simulink model "BrowarModel"  (R2024a)
settings: Solver=ode5  StartTime=0.0  StopTime=inf  FixedStep=0.1  RelTol=1e-3
undefined symbols (not defined in the file or in its folder): localhost, Matrikon, OI
libraries: opclib x24
(part 4 of 9)

== system BrowarModel/System dozowania drozdzy/XT806H ==
  note: Przetwornik pomiarowy
  In : Inport
  FT : Constant  Value=0
  FT_value : Constant  Value=0
  GUIMon : Gain
  Switch : Switch  Threshold=0.5  SaturateOnIntegerOverflow=off  InputSameDT=off
  Out : Outport
  wires:
  FT_value/1 -> Switch/1
  Switch/1 -> GUIMon/1
  FT/1 -> Switch/2
  GUIMon/1 -> Out/1
  In/1 -> Switch/3

== system BrowarModel/System dozowania drozdzy/XT806L ==
  note: Przetwornik pomiarowy
  In : Inport
  FT : Constant  Value=0
  FT_value : Constant  Value=0
  GUIMon : Gain
  Switch : Switch  Threshold=0.5  SaturateOnIntegerOverflow=off  InputSameDT=off
  Out : Outport
  wires:
  In/1 -> Switch/3
  GUIMon/1 -> Out/1
  FT/1 -> Switch/2
  Switch/1 -> GUIMon/1
  FT_value/1 -> Switch/1

== system BrowarModel/System dozowania drozdzy/XV804 ==
  note: Sterowanie
  GUIMon : Gain
  Lokalne : Constant  Value=0
  Wybor : Switch  Threshold=0.5  SaturateOnIntegerOverflow=off  InputSameDT=off
  Out : Outport
  wires:
  GUIMon/1 -> Out/1
  Wybor/1 -> GUIMon/1
  [TrybSter] -> Wybor/2
  [XV804] -> Wybor/1
  Lokalne/1 -> Wybor/3

== system BrowarModel/System dozowania drozdzy/XV806 ==
  note: Sterowanie
  GUIMon : Gain
  Lokalne : Constant  Value=0
  Wybor : Switch  Threshold=0.5  SaturateOnIntegerOverflow=off  InputSameDT=off
  Out : Outport
  wires:
  Lokalne/1 -> Wybor/3
  [XV806] -> Wybor/1
  [TrybSter] -> Wybor/2
  Wybor/1 -> GUIMon/1
  GUIMon/1 -> Out/1

== system BrowarModel/Kadz fermentacyjna/ET704/Zaklocenia pomiarowe ==
  Product1 : Product  InputSameDT=on  RndMeth=Zero  SaturateOnIntegerOverflow=on  OutDataTypeStr=Inherit: Same as first input
  Product3 : Product  InputSameDT=on  RndMeth=Zero  SaturateOnIntegerOverflow=on  OutDataTypeStr=Inherit: Same as first input
  Random Number : RandomNumber  Variance=.5  Seed=4365624  SampleTime=0.1
  Transfer Fcn1 : TransferFcn  Denominator=[0.5 1]
  Transfer Fcn2 : TransferFcn  Denominator=[0.5 1]
  Zaklocenia pomiarowe : Constant  Value=ZakloceniaPom
  Out : Outport
  wires:
  Random Number/1 -> Product3/1
  Product3/1 -> Transfer Fcn1/1
  Transfer Fcn1/1 -> Transfer Fcn2/1
  Transfer Fcn2/1 -> Out/1
  Zaklocenia pomiarowe/1 -> Product1/2
  [ZaklPom] -> Product1/1
  Product1/1 -> Product3/2

== system BrowarModel/Kadz fermentacyjna/ET705/Zaklocenia pomiarowe ==
  Product1 : Product  InputSameDT=on  RndMeth=Zero  SaturateOnIntegerOverflow=on  OutDataTypeStr=Inherit: Same as first input
  Product3 : Product  InputSameDT=on  RndMeth=Zero  SaturateOnIntegerOverflow=on  OutDataTypeStr=Inherit: Same as first input
  Random Number : RandomNumber  Variance=.5  Seed=4365624  SampleTime=0.1
  Transfer Fcn1 : TransferFcn  Denominator=[0.5 1]
  Transfer Fcn2 : TransferFcn  Denominator=[0.5 1]
  Zaklocenia pomiarowe : Constant  Value=ZakloceniaPom
  Out : Outport
  wires:
  Product1/1 -> Product3/2
  [ZaklPom] -> Product1/1
  Zaklocenia pomiarowe/1 -> Product1/2
  Transfer Fcn2/1 -> Out/1
  Transfer Fcn1/1 -> Transfer Fcn2/1
  Product3/1 -> Transfer Fcn1/1
  Random Number/1 -> Product3/1

== system BrowarModel/Kadz fermentacyjna/Kadz fermentacyjna/Kadz ==
  note: Kadz fermentacji
  Doplyw brzeczki : Inport
  Odplyw : Inport  Port=2
  Strumien ciepla : Inport  Port=3
  Temperatura brzeczki : Inport  Port=4
  Wyciek : Inport  Port=5
  Obroty mieszadla : Inport  Port=6
  Gain : Gain  Gain=1/1.5
  Math Function : Math  Operator=sqrt  SignedPower=on
  Max wyciek : Constant  Value=0.1
  Model akumulacji ciepla w zbiorniku z ciecza : Subsystem
  Model rozkladu temperatur : Subsystem
  Model utratu ciepla : Subsystem
  Objetosc : Integrator  InitialCondition=0.001  LimitOutput=on  UpperSaturationLimit=48  LowerSaturationLimit=0.001
  Powierzchnia dna m2 : Constant  Value=16
  Poziom zbiornika : Subsystem
  Product : Product  RndMeth=Zero
  Product1 : Product  RndMeth=Zero
  Sat doplyw (F>=0) : Saturate  UpperLimit=inf  LowerLimit=0
  Sat uszk (F>=0)1 : Saturate  UpperLimit=1  LowerLimit=0
  Sum1 : Sum  Inputs=|+-
  Sum2 : Sum  Inputs=|+-
  Sum4 : Sum  Inputs=|++
  Poziom wysoki : Outport
  Poziom niski : Outport  Port=2
  Poziom : Outport  Port=3
  Temp sensor gorny : Outport  Port=4
  Temp sensor srodkowy : Outport  Port=5
  Temp sensor dolny : Outport  Port=6
  Cieplo odebrane : Outport  Port=7
  Temperatura srednia : Outport  Port=8
  Temp przy dnie : Outport  Port=9
  wires:
  Model rozkladu temperatur/1(Temperatura lustra zbiornika) -> Model utratu ciepla/4(Temperatura lustra)  "dec C"
  Model utratu ciepla/1(Strumien ciepla) -> Model akumulacji ciepla w zbiorniku z ciecza/5(Strumien cieplo traconego)
  Sat doplyw (F>=0)/1 -> Sum1/1, Model akumulacji ciepla w zbiorniku z ciecza/3(Strumien doplywu cieczy)  "m3/s"
  Model akumulacji ciepla w zbiorniku z ciecza/2(Srednia temperaturacie czy) -> Model rozkladu temperatur/2(Srednia temperatura), Model utratu ciepla/3(Srednia temperatura), Temperatura srednia/1
  Powierzchnia dna m2/1 -> Model utratu ciepla/2(Pole podstawy zbiornika), Poziom zbiornika/2(Powierzchnia dna)  "m2"
  Objetosc/1 -> Model akumulacji ciepla w zbiorniku z ciecza/1(Objetosc cieczy w zbiorniku), Poziom zbiornika/1(Objetosc)  "m3"
  Poziom zbiornika/3(Poziom) -> Model utratu ciepla/1(Poziom), Poziom/1, Model rozkladu temperatur/1(Poziom), Gain/1
  Sum2/1 -> Objetosc/1
  Sum1/1 -> Sum2/1
  Model akumulacji ciepla w zbiorniku z ciecza/1(Srumien cieczy odparowanej) -> Sum2/2  "m3/s"
  Poziom zbiornika/1(Poziom  wysoki) -> Poziom wysoki/1
  Doplyw brzeczki/1 -> Sat doplyw (F>=0)/1
  Poziom zbiornika/2(Poziom niski) -> Poziom niski/1
  Model rozkladu temperatur/2(Sensor temperatury gorny) -> Temp sensor gorny/1
  Model rozkladu temperatur/3(Sensor temperatury srodkowy) -> Temp sensor srodkowy/1
  Model rozkladu temperatur/4(Sensor temperatury dolny) -> Temp sensor dolny/1
  Obroty mieszadla/1 -> Model rozkladu temperatur/3(Obroty mieszadla)
  Strumien ciepla/1 -> Model akumulacji ciepla w zbiorniku z ciecza/4(Strumien cieplna dostepny)
  Model rozkladu temperatur/5(Temperatura przy dnie zbiornika) -> Temp przy dnie/1
  Model akumulacji ciepla w zbiorniku z ciecza/3(Strumien ciepla odebrany) -> Cieplo odebrane/1
  Temperatura brzeczki/1 -> Model akumulacji ciepla w zbiorniku z ciecza/6(Temperatura strumien doplywu cieczy)
  Odplyw/1 -> Sum4/1  "m3/h"
  Wyciek/1 -> Sat uszk (F>=0)1/1
  Product/1 -> Sum4/2
  Sat uszk (F>=0)1/1 -> Product/1
  Product1/1 -> Product/2
  Max wyciek/1 -> Product1/1  "m3/s"
  Math Function/1 -> Product1/2
  Gain/1 -> Math Function/1
  Sum4/1 -> Sum1/2, Model akumulacji ciepla w zbiorniku z ciecza/2(Strumien odplywu cieczy)

== system BrowarModel/Kadz fermentacyjna/Kadz fermentacyjna/Model mieszadla ==
  Poziom : Inport
  Obroty : Inport  Port=2
  " Redukcja obrotow" : Gain  Gain=1/720
  " Redukcja obrotow1" : Gain  Gain=1/4
  Dot Product : DotProduct  OutDataTypeStr=Inherit: Inherit via internal rule
  Math Function : Math  Operator=square  SignedPower=on
  Sat FS : Saturate  UpperLimit=1  LowerLimit=0
  Wplyw stopnia wypelnienia na obciazenie : Lookup  InputValues=[0,0.3,1,2]  Table=[0.1,0.1,1,1]  SaturateOnIntegerOverflow=off
  Obroty zredukowane : Outport
  Obciazenie : Outport  Port=2
  wires:
  Obroty/1 -> " Redukcja obrotow"/1  "obr/min"
  " Redukcja obrotow"/1 -> Math Function/1, Obroty zredukowane/1  "obr/min"
  Poziom/1 -> Wplyw stopnia wypelnienia na obciazenie/1
  Math Function/1 -> " Redukcja obrotow1"/1
  " Redukcja obrotow1"/1 -> Dot Product/1
  Wplyw stopnia wypelnienia na obciazenie/1 -> Dot Product/2
  Dot Product/1 -> Sat FS/1
  Sat FS/1 -> Obciazenie/1

== system BrowarModel/Kadz fermentacyjna/Kadz fermentacyjna/Model ogrzewacza ==
  note: Ogrzewacz elektryczny
  note: Uszkodzenie ogrzewacza
  Sterowanie : Inport
  Spadek mocy : Inport  Port=2
  Const : Constant  Value=100
  GUIMon : Gain
  Gain : Gain  Gain=1/100
  Gain1 : Gain  Gain=1/100
  Maksymalna moc : Constant  Value=10000000
  Product : Product  RndMeth=Zero
  Product1 : Product  RndMeth=Zero
  Quantizer : Quantizer  QuantizationInterval=20
  Sat ster : Saturate  UpperLimit=100  LowerLimit=0
  Sat uszk : Saturate  UpperLimit=100  LowerLimit=0
  Sat zero : Saturate  UpperLimit=inf  LowerLimit=0
  Sum1 : Sum  Inputs=|+-
  Sum2 : Sum  Inputs=|+-
  Transfer Fcn : TransferFcn  Denominator=[60 1]
  Transfer Fcn1 : TransferFcn  Denominator=[60 1]
  Zaklocenia : Subsystem
  Cieplo dostarczone : Outport
  wires:
  Sat ster/1 -> Quantizer/1
  Sterowanie/1 -> Sat ster/1
  Quantizer/1 -> GUIMon/1
  Gain/1 -> Product/1
  Zaklocenia/1(Out) -> Sum1/2
  Product/1 -> Transfer Fcn/1
  Transfer Fcn/1 -> Transfer Fcn1/1
  Sum1/1 -> Sat zero/1
  Transfer Fcn1/1 -> Sum1/1, Zaklocenia/1(In)
  GUIMon/1 -> Gain/1
  Sat zero/1 -> Cieplo dostarczone/1
  Maksymalna moc/1 -> Product1/1
  Product1/1 -> Product/2
  Spadek mocy/1 -> Sat uszk/1
  Sat uszk/1 -> Sum2/2
  Sum2/1 -> Gain1/1
  Const/1 -> Sum2/1
  Gain1/1 -> Product1/2

== system BrowarModel/Kadz fermentacyjna/Kadz fermentacyjna/Odplyw z kadzi ==
  note: Doplyw kadzi
  Sterowanie zaworu : Inport
  Przeciek zaworu : Inport  Port=2
  Dlawienie zaworu : Inport  Port=3
  Wyciek : Inport  Port=4
  Poziom w kadzi : Inport  Port=5
  Zalaczenie pompy : Inport  Port=6
  Sterowanie pompy : Inport  Port=7
  Uszkodzenie pompy : Inport  Port=8
  Charakterystyka pompy : Lookup  InputValues="[0\t125\t250\t375\t500\t625\t750\t875\t1000\t1125\t1250\t1375\t1500 1625]"  Table=|  SaturateOnIntegerOverflow=off
      | [0 50	125	178	220	250	270	288	300	310	315	320	323	327
      | ]
  Gain : Gain  Gain=1/100
  Obciazenie silnika : Gain  Gain=1/500
  Product : Product  RndMeth=Zero
  Product1 : Product  RndMeth=Zero
  Relay : Relay  OnOutputValue=0  OffOutputValue=1
  Relay1 : Relay
  Sat uszk : Saturate  UpperLimit=100  LowerLimit=0
  Silnik elektryczny : Subsystem
  "Sterowanie " : DotProduct  OutDataTypeStr=Inherit: Inherit via internal rule
  Straty pompy : Gain  Gain=50/0.15
  Sum : Sum  Inputs=|+-
  Sum1 : Sum  Inputs=|+-
  Wplyw stopnia wypelnienia kadzi : Lookup  InputValues=[-1, 0, 0.05, 1]  Table=[0, 0, 1,1]  SaturateOnIntegerOverflow=off
  Wplyw uszkodzenia : Product  RndMeth=Zero
  Zawor dyskretny : Subsystem
  Przeplyw_wyciek : Outport
  Przeplyw : Outport  Port=2
  Obroty : Outport  Port=3
  Prad silnika : Outport  Port=4
  Silnik Idle : Outport  Port=5
  Silnik Running : Outport  Port=6
  Silnik Alarm : Outport  Port=7
  wires:
  Wplyw stopnia wypelnienia kadzi/1 -> Product/1  "[0,1]"
  Zawor dyskretny/1(Przeplyw) -> Sum1/1, Straty pompy/1, Product1/1
  Dlawienie zaworu/1 -> Zawor dyskretny/4(Dlawienie)
  Poziom w kadzi/1 -> Wplyw stopnia wypelnienia kadzi/1  "m"
  Zalaczenie pompy/1 -> Relay1/1, Silnik elektryczny/1(Zalaczenie)
  Uszkodzenie pompy/1 -> Relay/1, Silnik elektryczny/4(Uszkodzenie)
  Relay/1 -> Wplyw uszkodzenia/2
  Silnik elektryczny/1(Obroty) -> Charakterystyka pompy/1, Obroty/1
  Wplyw uszkodzenia/1 -> Product/2
  Charakterystyka pompy/1 -> "Sterowanie "/2  "kPa"
  "Sterowanie "/1 -> Wplyw uszkodzenia/1
  Relay1/1 -> "Sterowanie "/1
  Product/1 -> Sum/1, Obciazenie silnika/1
  Sum/1 -> Zawor dyskretny/2(Cisnienie)
  Straty pompy/1 -> Sum/2
  Wyciek/1 -> Sat uszk/1
  Product1/1 -> Przeplyw_wyciek/1, Sum1/2
  Sum1/1 -> Przeplyw/1
  Sat uszk/1 -> Gain/1
  Przeciek zaworu/1 -> Zawor dyskretny/3(Przeciek)
  Sterowanie zaworu/1 -> Zawor dyskretny/1(Sterowanie)
  Gain/1 -> Product1/2
  Silnik elektryczny/2(Prad) -> Prad silnika/1
  Silnik elektryczny/3(Idle) -> Silnik Idle/1
  Silnik elektryczny/4(Running) -> Silnik Running/1
  Silnik elektryczny/5(Alarm) -> Silnik Alarm/1
  Sterowanie pompy/1 -> Silnik elektryczny/2(Zadane obroty)
  Obciazenie silnika/1 -> Silnik elektryczny/3(Obciazenie zew)

== system BrowarModel/Kadz fermentacyjna/Kadz fermentacyjna/Silnik elektryczny ==
  note: Uszkodzenie silnika
  note: Silnik elektryczny
  Zalaczenie : Inport
  Zadane obroty : Inport  Port=2
  Obciazenie zew : Inport  Port=3
  Uszkodzenie : Inport  Port=4
  Abs : Abs  SaturateOnIntegerOverflow=off
  Add : Sum
  Add1 : Sum  Inputs=+-
  Const : Constant
  Gain : Gain
  "Hz -> obr/min" : Gain  Gain=60/2
  Inercja mechaniczna : TransferFcn  Denominator=[1 1]
  Poslizg : DotProduct  OutDataTypeStr=Inherit: Inherit via internal rule
  Poslizg jalowy : Constant  Value=0.04
  Poslizg od obciazenia : Gain  Gain=0.05
  Prad jalowy : Gain  Gain=0.5
  Prad nominalny (10A) : Constant  Value=10
  Relay : Relay  OnOutputValue=0  OffOutputValue=1
  Saturation [0,1] : Saturate  UpperLimit=1  LowerLimit=0
  "Saturation [0,1] " : Saturate  UpperLimit=1  LowerLimit=0
  Stan : Subsystem
  Sterowanie : Subsystem
  Sterownik : Subsystem
  Sum : Sum  Inputs=|+-
  Sum1 : Sum  Inputs=|++
  Sum2 : Sum  Inputs=|+-
  Sum3 : Sum  Inputs=|++
  Wplyw uszkodzenia : DotProduct  OutDataTypeStr=Inherit: Inherit via internal rule
  Wplyw obciazenia : DotProduct  OutDataTypeStr=Inherit: Inherit via internal rule
  Wplyw obrotow : DotProduct  OutDataTypeStr=Inherit: Inherit via internal rule
  Zaklocenia : Subsystem
  Zalaczony : DotProduct  OutDataTypeStr=Inherit: Inherit via internal rule
  "obr/min -> FS  " : Gain  Gain=1/1500
  "obr/min -> Hz" : Gain  Gain=1/60*2
  Obroty : Outport
  Prad : Outport  Port=2
  Idle : Outport  Port=3
  Running : Outport  Port=4
  Alarm : Outport  Port=5
  wires:
  Zaklocenia/1(Out) -> Sum2/2
  Sum2/1 -> Sum/1, Add1/1
  Stan/3(Alarm) -> Alarm/1
  Stan/2(Running) -> Zalaczony/2, Running/1
  Stan/1(Idle) -> Idle/1
  Zadane obroty/1 -> Sterowanie/1(Zadane obroty)
  Zalaczony/1 -> Wplyw obrotow/2
  Sum1/1 -> Zalaczony/1  "A"
  Wplyw obrotow/1 -> Prad/1  "A"
  Wplyw uszkodzenia/1 -> "Hz -> obr/min"/1
  Relay/1 -> Stan/2(Zdatny), Wplyw uszkodzenia/2
  Sterownik/1(CV) -> Wplyw uszkodzenia/1
  Uszkodzenie/1 -> Relay/1
  Gain/1 -> "Saturation [0,1] "/1
  Sterowanie/1(Sterowanie) -> Sterownik/2(SP)
  Zalaczenie/1 -> Stan/1(Zalaczony), Sterowanie/2(Zalaczenie)
  "Saturation [0,1] "/1 -> Add/1
  "obr/min -> FS  "/1 -> Gain/1
  Add1/1 -> "obr/min -> FS  "/1
  Add/1 -> Abs/1, Poslizg od obciazenia/1  "FS"
  Saturation [0,1]/1 -> Add/2
  "obr/min -> Hz"/1 -> Sterownik/1(PV)
  Const/1 -> Wplyw obrotow/1
  Abs/1 -> Wplyw obciazenia/1  "FS"
  Wplyw obciazenia/1 -> Sum1/1
  Prad jalowy/1 -> Wplyw obciazenia/2, Sum1/2
  Prad nominalny (10A)/1 -> Prad jalowy/1  "A"
  Poslizg jalowy/1 -> Sum3/2
  Obciazenie zew/1 -> Saturation [0,1]/1  "FS"
  Poslizg od obciazenia/1 -> Sum3/1
  Sum3/1 -> Poslizg/2
  Poslizg/1 -> Sum/2
  "Hz -> obr/min"/1 -> Zaklocenia/1(In), Sum2/1  "[obr/min]"
  Sum/1 -> Inercja mechaniczna/1
  Inercja mechaniczna/1 -> "obr/min -> Hz"/1, Add1/2, Poslizg/1, Obroty/1

== system BrowarModel/Kadz fermentacyjna/LT701/Zaklocenia pomiarowe ==
  Product1 : Product  InputSameDT=on  RndMeth=Zero  SaturateOnIntegerOverflow=on  OutDataTypeStr=Inherit: Same as first input
  Product3 : Product  InputSameDT=on  RndMeth=Zero  SaturateOnIntegerOverflow=on  OutDataTypeStr=Inherit: Same as first input
  Random Number : RandomNumber  Variance=.5  Seed=4365624  SampleTime=0.1
  Transfer Fcn1 : TransferFcn  Denominator=[0.5 1]
  Transfer Fcn2 : TransferFcn  Denominator=[0.5 1]
  Zaklocenia pomiarowe : Constant  Value=ZakloceniaPom
  Out : Outport
  wires:
  Product1/1 -> Product3/2
  [ZaklPom] -> Product1/1
  Zaklocenia pomiarowe/1 -> Product1/2
  Transfer Fcn2/1 -> Out/1
  Transfer Fcn1/1 -> Transfer Fcn2/1
  Product3/1 -> Transfer Fcn1/1
  Random Number/1 -> Product3/1

== system BrowarModel/Kadz fermentacyjna/ST704/Zaklocenia pomiarowe ==
  Product1 : Product  InputSameDT=on  RndMeth=Zero  SaturateOnIntegerOverflow=on  OutDataTypeStr=Inherit: Same as first input
  Product3 : Product  InputSameDT=on  RndMeth=Zero  SaturateOnIntegerOverflow=on  OutDataTypeStr=Inherit: Same as first input
  Random Number : RandomNumber  Variance=.5  Seed=4365624  SampleTime=0.1
  Transfer Fcn1 : TransferFcn  Denominator=[0.5 1]
  Transfer Fcn2 : TransferFcn  Denominator=[0.5 1]
  Zaklocenia pomiarowe : Constant  Value=ZakloceniaPom
  Out : Outport
  wires:
  Product1/1 -> Product3/2
  [ZaklPom] -> Product1/1
  Zaklocenia pomiarowe/1 -> Product1/2
  Transfer Fcn2/1 -> Out/1
  Transfer Fcn1/1 -> Transfer Fcn2/1
  Product3/1 -> Transfer Fcn1/1
  Random Number/1 -> Product3/1

== system BrowarModel/Kadz fermentacyjna/ST705/Zaklocenia pomiarowe ==
  Product1 : Product  InputSameDT=on  RndMeth=Zero  SaturateOnIntegerOverflow=on  OutDataTypeStr=Inherit: Same as first input
  Product3 : Product  InputSameDT=on  RndMeth=Zero  SaturateOnIntegerOverflow=on  OutDataTypeStr=Inherit: Same as first input
  Random Number : RandomNumber  Variance=.5  Seed=4365624  SampleTime=0.1
  Transfer Fcn1 : TransferFcn  Denominator=[0.5 1]
  Transfer Fcn2 : TransferFcn  Denominator=[0.5 1]
  Zaklocenia pomiarowe : Constant  Value=ZakloceniaPom
  Out : Outport
  wires:
  Random Number/1 -> Product3/1
  Product3/1 -> Transfer Fcn1/1
  Transfer Fcn1/1 -> Transfer Fcn2/1
  Transfer Fcn2/1 -> Out/1
  Zaklocenia pomiarowe/1 -> Product1/2
  [ZaklPom] -> Product1/1
  Product1/1 -> Product3/2

== system BrowarModel/Kadz fermentacyjna/TT702H/Zaklocenia pomiarowe ==
  Product1 : Product  InputSameDT=on  RndMeth=Zero  SaturateOnIntegerOverflow=on  OutDataTypeStr=Inherit: Same as first input
  Product3 : Product  InputSameDT=on  RndMeth=Zero  SaturateOnIntegerOverflow=on  OutDataTypeStr=Inherit: Same as first input
  Random Number : RandomNumber  Variance=.5  Seed=4365624  SampleTime=0.1
  Transfer Fcn1 : TransferFcn  Denominator=[0.5 1]
  Transfer Fcn2 : TransferFcn  Denominator=[0.5 1]
  Zaklocenia pomiarowe : Constant  Value=ZakloceniaPom
  Out : Outport
  wires:
  Random Number/1 -> Product3/1
  Product3/1 -> Transfer Fcn1/1
  Transfer Fcn1/1 -> Transfer Fcn2/1
  Transfer Fcn2/1 -> Out/1
  Zaklocenia pomiarowe/1 -> Product1/2
  [ZaklPom] -> Product1/1
  Product1/1 -> Product3/2

== system BrowarModel/Kadz fermentacyjna/TT702L/Zaklocenia pomiarowe ==
  Product1 : Product  InputSameDT=on  RndMeth=Zero  SaturateOnIntegerOverflow=on  OutDataTypeStr=Inherit: Same as first input
  Product3 : Product  InputSameDT=on  RndMeth=Zero  SaturateOnIntegerOverflow=on  OutDataTypeStr=Inherit: Same as first input
  Random Number : RandomNumber  Variance=.5  Seed=4365624  SampleTime=0.1
  Transfer Fcn1 : TransferFcn  Denominator=[0.5 1]
  Transfer Fcn2 : TransferFcn  Denominator=[0.5 1]
  Zaklocenia pomiarowe : Constant  Value=ZakloceniaPom
  Out : Outport
  wires:
  Random Number/1 -> Product3/1
  Product3/1 -> Transfer Fcn1/1
  Transfer Fcn1/1 -> Transfer Fcn2/1
  Transfer Fcn2/1 -> Out/1
  Zaklocenia pomiarowe/1 -> Product1/2
  [ZaklPom] -> Product1/1
  Product1/1 -> Product3/2

== system BrowarModel/Kadz fermentacyjna/TT702M/Zaklocenia pomiarowe ==
  Product1 : Product  InputSameDT=on  RndMeth=Zero  SaturateOnIntegerOverflow=on  OutDataTypeStr=Inherit: Same as first input
  Product3 : Product  InputSameDT=on  RndMeth=Zero  SaturateOnIntegerOverflow=on  OutDataTypeStr=Inherit: Same as first input
  Random Number : RandomNumber  Variance=.5  Seed=4365624  SampleTime=0.1
  Transfer Fcn1 : TransferFcn  Denominator=[0.5 1]
  Transfer Fcn2 : TransferFcn  Denominator=[0.5 1]
  Zaklocenia pomiarowe : Constant  Value=ZakloceniaPom
  Out : Outport
  wires:
  Product1/1 -> Product3/2
  [ZaklPom] -> Product1/1
  Zaklocenia pomiarowe/1 -> Product1/2
  Transfer Fcn2/1 -> Out/1
  Transfer Fcn1/1 -> Transfer Fcn2/1
  Product3/1 -> Transfer Fcn1/1
  Random Number/1 -> Product3/1

== system BrowarModel/Kadz filtracji/ET302/Zaklocenia pomiarowe ==
  Product1 : Product  InputSameDT=on  RndMeth=Zero  SaturateOnIntegerOverflow=on  OutDataTypeStr=Inherit: Same as first input
  Product3 : Product  InputSameDT=on  RndMeth=Zero  SaturateOnIntegerOverflow=on  OutDataTypeStr=Inherit: Same as first input
  Random Number : RandomNumber  Variance=.5  Seed=4365624  SampleTime=0.1
  Transfer Fcn1 : TransferFcn  Denominator=[0.5 1]
  Transfer Fcn2 : TransferFcn  Denominator=[0.5 1]
  Zaklocenia pomiarowe : Constant  Value=ZakloceniaPom
  Out : Outport
  wires:
  Random Number/1 -> Product3/1
  Product3/1 -> Transfer Fcn1/1
  Transfer Fcn1/1 -> Transfer Fcn2/1
  Transfer Fcn2/1 -> Out/1
  Zaklocenia pomiarowe/1 -> Product1/2
  [ZaklPom] -> Product1/1
  Product1/1 -> Product3/2

== system BrowarModel/Kadz filtracji/ET304/Zaklocenia pomiarowe ==
  Product1 : Product  InputSameDT=on  RndMeth=Zero  SaturateOnIntegerOverflow=on  OutDataTypeStr=Inherit: Same as first input
  Product3 : Product  InputSameDT=on  RndMeth=Zero  SaturateOnIntegerOverflow=on  OutDataTypeStr=Inherit: Same as first input
  Random Number : RandomNumber  Variance=.5  Seed=4365624  SampleTime=0.1
  Transfer Fcn1 : TransferFcn  Denominator=[0.5 1]
  Transfer Fcn2 : TransferFcn  Denominator=[0.5 1]
  Zaklocenia pomiarowe : Constant  Value=ZakloceniaPom
  Out : Outport
  wires:
  Product1/1 -> Product3/2
  [ZaklPom] -> Product1/1
  Zaklocenia pomiarowe/1 -> Product1/2
  Transfer Fcn2/1 -> Out/1
  Transfer Fcn1/1 -> Transfer Fcn2/1
  Product3/1 -> Transfer Fcn1/1
  Random Number/1 -> Product3/1

== system BrowarModel/Kadz filtracji/ET307/Zaklocenia pomiarowe ==
  Product1 : Product  InputSameDT=on  RndMeth=Zero  SaturateOnIntegerOverflow=on  OutDataTypeStr=Inherit: Same as first input
  Product3 : Product  InputSameDT=on  RndMeth=Zero  SaturateOnIntegerOverflow=on  OutDataTypeStr=Inherit: Same as first input
  Random Number : RandomNumber  Variance=.5  Seed=4365624  SampleTime=0.1
  Transfer Fcn1 : TransferFcn  Denominator=[0.5 1]
  Transfer Fcn2 : TransferFcn  Denominator=[0.5 1]
  Zaklocenia pomiarowe : Constant  Value=ZakloceniaPom
  Out : Outport
  wires:
  Product1/1 -> Product3/2
  [ZaklPom] -> Product1/1
  Zaklocenia pomiarowe/1 -> Product1/2
  Transfer Fcn2/1 -> Out/1
  Transfer Fcn1/1 -> Transfer Fcn2/1
  Product3/1 -> Transfer Fcn1/1
  Random Number/1 -> Product3/1

== system BrowarModel/Kadz filtracji/Kadz filtracji/Doplyw kadzi ==
  note: Doplyw kadzi
  Sterowanie zaworu : Inport
  Przeciek zaworu : Inport  Port=2
  Dlawienie zaworu : Inport  Port=3
  Wyciek : Inport  Port=4
  Poziom w kadzi zaciernej : Inport  Port=5
  Zalaczenie pompy : Inport  Port=6
  Sterowanie pompy : Inport  Port=7
  Uszkodzenie pompy : Inport  Port=8
  Przepelnienire zb gorny : Inport  Port=9
  Charakterystyka pompy : Lookup  InputValues="[0\t125\t250\t375\t500\t625\t750\t875\t1000\t1125\t1250\t1375\t1500 1625]"  Table=|  SaturateOnIntegerOverflow=off
      | [0 50	125	178	220	250	270	288	300	310	315	320	323	327
      | ]
  Constant : Constant  Value=0
  Gain : Gain  Gain=1/100
  Obciazenie silnika : Gain  Gain=1/500
  Product : Product  RndMeth=Zero
  Product1 : Product  RndMeth=Zero
  Relay : Relay  OnOutputValue=0  OffOutputValue=1
  Relay1 : Relay
  Sat uszk : Saturate  UpperLimit=100  LowerLimit=0
  Silnik elektryczny : Subsystem
  "Sterowanie " : DotProduct  OutDataTypeStr=Inherit: Inherit via internal rule
  Straty pompy : Gain  Gain=50/0.15
  Sum : Sum  Inputs=|+-
  Sum1 : Sum  Inputs=|+-
  Switch : Switch  Threshold=0.5  SaturateOnIntegerOverflow=off  InputSameDT=off
  Wplyw stopnia wypelnienia kadzi zaciernej : Lookup  InputValues=[-1, 0, 0.001, 0.05, 1]  Table=[0, 0, 0, 1, 1]  SaturateOnIntegerOverflow=off
  Wplyw uszkodzenia : Product  RndMeth=Zero
  Zawor dyskretny : Subsystem
  Przeplyw : Outport
  Przeplyw_wyciek : Outport  Port=2
  Obroty : Outport  Port=3
  Prad silnika : Outport  Port=4
  Silnik Idle : Outport  Port=5
  Silnik Running : Outport  Port=6
  Silnik Alarm : Outport  Port=7
  wires:
  Wplyw stopnia wypelnienia kadzi zaciernej/1 -> Product/1  "[0,1]"
  Zawor dyskretny/1(Przeplyw) -> Sum1/1, Straty pompy/1, Product1/1
  Dlawienie zaworu/1 -> Zawor dyskretny/4(Dlawienie)
  Poziom w kadzi zaciernej/1 -> Wplyw stopnia wypelnienia kadzi zaciernej/1  "m"
  Zalaczenie pompy/1 -> Relay1/1, Silnik elektryczny/1(Zalaczenie)
  Uszkodzenie pompy/1 -> Relay/1, Silnik elektryczny/4(Uszkodzenie)
  Relay/1 -> Wplyw uszkodzenia/2
  Silnik elektryczny/1(Obroty) -> Charakterystyka pompy/1, Obroty/1
  Wplyw uszkodzenia/1 -> Product/2
  Charakterystyka pompy/1 -> "Sterowanie "/2  "kPa"
  "Sterowanie "/1 -> Wplyw uszkodzenia/1
  Relay1/1 -> "Sterowanie "/1
  Product/1 -> Sum/1, Obciazenie silnika/1
  Sum/1 -> Zawor dyskretny/2(Cisnienie)
  Straty pompy/1 -> Sum/2
  Wyciek/1 -> Sat uszk/1
  Product1/1 -> Przeplyw_wyciek/1, Sum1/2
  Sat uszk/1 -> Gain/1
  Przeciek zaworu/1 -> Zawor dyskretny/3(Przeciek)
  Sterowanie zaworu/1 -> Zawor dyskretny/1(Sterowanie)
  Gain/1 -> Product1/2
  Silnik elektryczny/2(Prad) -> Prad silnika/1
  Silnik elektryczny/3(Idle) -> Silnik Idle/1
  Silnik elektryczny/4(Running) -> Silnik Running/1
  Silnik elektryczny/5(Alarm) -> Silnik Alarm/1
  Sterowanie pompy/1 -> Silnik elektryczny/2(Zadane obroty)
  Obciazenie silnika/1 -> Silnik elektryczny/3(Obciazenie zew)
  Przepelnienire zb gorny/1 -> Switch/2
  Constant/1 -> Switch/1
  Sum1/1 -> Switch/3
  Switch/1 -> Przeplyw/1

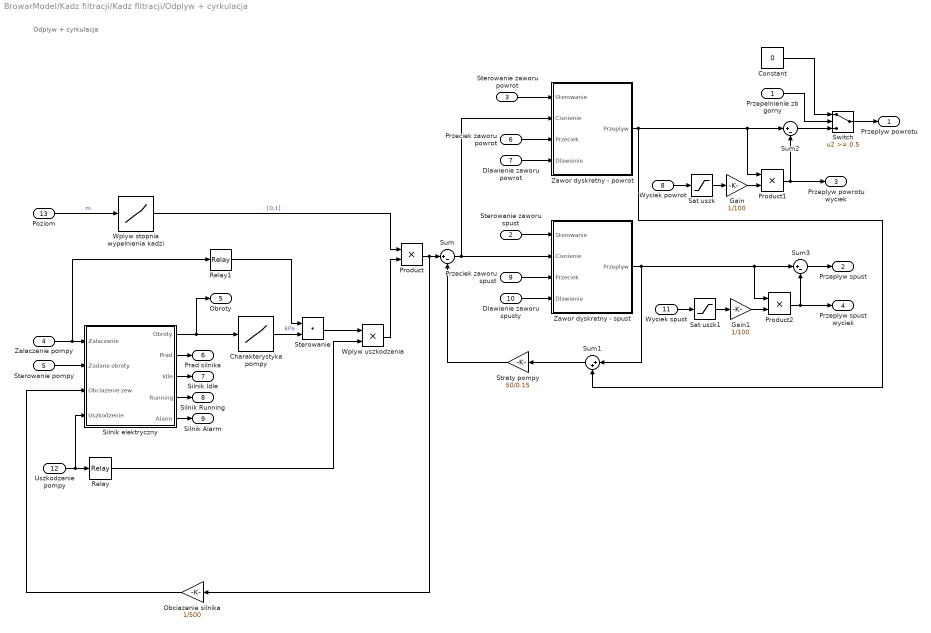
== system BrowarModel/Kadz filtracji/Kadz filtracji/Odplyw + cyrkulacja ==
  note: Odplyw + cyrkulacja
  Przepelnienie zb gorny : Inport
  Sterowanie zaworu spust : Inport  Port=2
  Sterowanie zaworu powrot : Inport  Port=3
  Zalaczenie pompy : Inport  Port=4
  Sterowanie pompy : Inport  Port=5
  Przeciek zaworu powrot : Inport  Port=6
  Dlawienie zaworu powrot : Inport  Port=7
  Wyciek powrot : Inport  Port=8
  Przeciek zaworu spust : Inport  Port=9
  Dlawienie zaworu spusty : Inport  Port=10
  Wyciek spust : Inport  Port=11
  Uszkodzenie pompy : Inport  Port=12
  Poziom : Inport  Port=13
  Charakterystyka pompy : Lookup  InputValues="[0\t125\t250\t375\t500\t625\t750\t875\t1000\t1125\t1250\t1375\t1500 1625]"  Table=|  SaturateOnIntegerOverflow=off
      | [0 50	125	178	220	250	270	288	300	310	315	320	323	327
      | ]
  Constant : Constant  Value=0
  Gain : Gain  Gain=1/100
  Gain1 : Gain  Gain=1/100
  Obciazenie silnika : Gain  Gain=1/500
  Product : Product  RndMeth=Zero
  Product1 : Product  RndMeth=Zero
  Product2 : Product  RndMeth=Zero
  Relay : Relay  OnOutputValue=0  OffOutputValue=1
  Relay1 : Relay
  Sat uszk : Saturate  UpperLimit=100  LowerLimit=0
  Sat uszk1 : Saturate  UpperLimit=100  LowerLimit=0
  Silnik elektryczny : Subsystem
  "Sterowanie " : DotProduct  OutDataTypeStr=Inherit: Inherit via internal rule
  Straty pompy : Gain  Gain=50/0.15
  Sum : Sum  Inputs=|+-
  Sum1 : Sum  Inputs=|++
  Sum2 : Sum  Inputs=|+-
  Sum3 : Sum  Inputs=|+-
  Switch : Switch  Threshold=0.5  SaturateOnIntegerOverflow=off  InputSameDT=off
  Wplyw stopnia wypelnienia kadzi : Lookup  InputValues=[-1, 0, 0.001 0.05, 1]  Table=[0, 0, 0, 1,1]  SaturateOnIntegerOverflow=off
  Wplyw uszkodzenia : Product  RndMeth=Zero
  Zawor dyskretny - powrot : Subsystem
  Zawor dyskretny - spust : Subsystem
  Przeplyw powrotu : Outport
  Przeplyw spust : Outport  Port=2
  Przeplyw powrotu wyciek : Outport  Port=3
  Przeplyw spust wyciek : Outport  Port=4
  Obroty : Outport  Port=5
  Prad silnika : Outport  Port=6
  Silnik Idle : Outport  Port=7
  Silnik Running : Outport  Port=8
  Silnik Alarm : Outport  Port=9
  wires:
  Sum/1 -> Zawor dyskretny - spust/2(Cisnienie), Zawor dyskretny - powrot/2(Cisnienie)
  Relay1/1 -> "Sterowanie "/1
  "Sterowanie "/1 -> Wplyw uszkodzenia/1
  Wplyw uszkodzenia/1 -> Product/2
  Relay/1 -> Wplyw uszkodzenia/2
  Uszkodzenie pompy/1 -> Relay/1, Silnik elektryczny/4(Uszkodzenie)
  Sterowanie pompy/1 -> Silnik elektryczny/2(Zadane obroty)
  Zalaczenie pompy/1 -> Relay1/1, Silnik elektryczny/1(Zalaczenie)
  Poziom/1 -> Wplyw stopnia wypelnienia kadzi/1  "m"
  Dlawienie zaworu spusty/1 -> Zawor dyskretny - spust/4(Dlawienie)
  Przeciek zaworu spust/1 -> Zawor dyskretny - spust/3(Przeciek)
  Zawor dyskretny - spust/1(Przeplyw) -> Sum1/1, Sum3/1, Product2/1
  Sterowanie zaworu spust/1 -> Zawor dyskretny - spust/1(Sterowanie)
  Wplyw stopnia wypelnienia kadzi/1 -> Product/1  "[0,1]"
  Dlawienie zaworu powrot/1 -> Zawor dyskretny - powrot/4(Dlawienie)
  Przeciek zaworu powrot/1 -> Zawor dyskretny - powrot/3(Przeciek)
  Zawor dyskretny - powrot/1(Przeplyw) -> Sum1/2, Sum2/1, Product1/1
  Sterowanie zaworu powrot/1 -> Zawor dyskretny - powrot/1(Sterowanie)
  Product/1 -> Sum/1, Obciazenie silnika/1
  Sum1/1 -> Straty pompy/1
  Straty pompy/1 -> Sum/2
  Product1/1 -> Przeplyw powrotu wyciek/1, Sum2/2
  Sat uszk/1 -> Gain/1
  Wyciek powrot/1 -> Sat uszk/1
  Sum3/1 -> Przeplyw spust/1
  Wyciek spust/1 -> Sat uszk1/1
  Sat uszk1/1 -> Gain1/1
  Product2/1 -> Sum3/2, Przeplyw spust wyciek/1
  Gain/1 -> Product1/2
  Gain1/1 -> Product2/2
  Silnik elektryczny/1(Obroty) -> Obroty/1, Charakterystyka pompy/1
  Charakterystyka pompy/1 -> "Sterowanie "/2  "kPa"
  Silnik elektryczny/2(Prad) -> Prad silnika/1
  Silnik elektryczny/3(Idle) -> Silnik Idle/1
  Silnik elektryczny/4(Running) -> Silnik Running/1
  Silnik elektryczny/5(Alarm) -> Silnik Alarm/1
  Obciazenie silnika/1 -> Silnik elektryczny/3(Obciazenie zew)
  Switch/1 -> Przeplyw powrotu/1
  Sum2/1 -> Switch/3
  Constant/1 -> Switch/1
  Przepelnienie zb gorny/1 -> Switch/2

== system BrowarModel/Kadz filtracji/Kadz filtracji/Zawor doplywu wody ==
  note: Zawor doplywu slodu
  note: Uszkodzenie:
      | Brak materialu
  note: Uszkodzenie:
      | Dlawienie przeplywu w zaworze
  note: Uszkodzenie:
      | Przeciek wewnetrzny w zaworze
  note: Uszkodzenie:
      | Wyciek zewnetrzny w zaworze
  Sterowanie : Inport
  Dlawienie : Inport  Port=2
  Przeciek : Inport  Port=3
  Wyciek : Inport  Port=4
  Brak : Inport  Port=5
  Const : Constant  Value=100
  Const1 : Constant  Value=100
  Const2 : Constant  Value=100
  Dead Zone : DeadZone  LowerValue=-inf  UpperValue=0.002
  GUIMon : Gain
  Gain : Gain  Gain=1/100
  Gain1 : Gain  Gain=1/100
  Gain2 : Gain  Gain=1/100
  Integer Delay : Delay  DelayLength=15
  Napelnianie m3/s : Gain  Gain=Fmax/100
  Product : Product  RndMeth=Zero
  Product1 : Product  RndMeth=Zero
  Product2 : Product  RndMeth=Zero
  Relay : Relay  OnOutputValue=100
  Sat (0-100) : Saturate  UpperLimit=100  LowerLimit=0
  Sat dlawienie (0-100) : Saturate  UpperLimit=100  LowerLimit=0
  Sat przecieku (0-100) : Saturate  UpperLimit=100  LowerLimit=0
  Sat uszk (0-100) : Saturate  UpperLimit=100  LowerLimit=0
  Sat wyciek (0-100) : Saturate  UpperLimit=100  LowerLimit=0
  Sum : Sum  Inputs=|+-
  Sum1 : Sum  Inputs=|++
  Sum2 : Sum  Inputs=|+-
  Sum3 : Sum  Inputs=|+-
  Sum5 : Sum  Inputs=|++
  Transfer Fcn : TransferFcn  Denominator=[1 1]
  Zaklocenia : Subsystem
  Przeplyw : Outport
  wires:
  Product/1 -> Transfer Fcn/1  "m3/s"
  Const/1 -> Sum/1
  Sat dlawienie (0-100)/1 -> Sum/2
  Sum/1 -> Gain/1
  Transfer Fcn/1 -> Integer Delay/1  "m3/s"
  Sterowanie/1 -> Relay/1
  Dlawienie/1 -> Sat dlawienie (0-100)/1  "[0,100]"
  Sat (0-100)/1 -> Napelnianie m3/s/1
  Sum1/1 -> Sat (0-100)/1
  Relay/1 -> GUIMon/1
  Przeciek/1 -> Sat przecieku (0-100)/1
  Sat przecieku (0-100)/1 -> Sum1/2
  Wyciek/1 -> Sat wyciek (0-100)/1
  Const1/1 -> Sum2/1
  Sat wyciek (0-100)/1 -> Sum2/2
  Integer Delay/1 -> Product1/1  "m3/s"
  Product1/1 -> Dead Zone/1
  Sum2/1 -> Gain1/1
  Gain1/1 -> Product1/2
  Product2/1 -> Sum1/1
  GUIMon/1 -> Product2/2
  Brak/1 -> Sat uszk (0-100)/1
  Const2/1 -> Sum3/1
  Sat uszk (0-100)/1 -> Sum3/2
  Sum3/1 -> Gain2/1
  Napelnianie m3/s/1 -> Sum5/1, Zaklocenia/1(In)
  Sum5/1 -> Product/2
  Gain/1 -> Product/1
  Zaklocenia/1(Out) -> Sum5/2
  Gain2/1 -> Product2/1
  Dead Zone/1 -> Przeplyw/1

== system BrowarModel/Kadz filtracji/Kadz filtracji/Zbiornik dolny ==
  note: Zbiornik dolny
  Doplyw zanieczyszczen : Inport
  Doplyw : Inport  Port=2
  Jakosc zacieru : Inport  Port=3
  Temperatura doplywu : Inport  Port=4
  Odplyw : Inport  Port=5
  Wyciek : Inport  Port=6
  Display1 : Display
  Divide1 : Product  Inputs=*/
  Dot Product : DotProduct  OutDataTypeStr=Inherit: Inherit via internal rule
  Gain : Gain  Gain=1/4
  Masa zanieczyszczen : Integrator  InitialCondition=0.001*0.2  LimitOutput=on  UpperSaturationLimit=48  LowerSaturationLimit=0.001*0.2
  Math Function : Math  Operator=sqrt  SignedPower=on
  Max wyciek : Constant  Value=0.1
  Model akumulacji ciepla w zbiorniku : Subsystem
  Model jakosci zacieru : Subsystem
  Model utratu ciepla : Subsystem
  Objetosc zbiornik dolny : Integrator  InitialCondition=0.001  LimitOutput=on  UpperSaturationLimit=48  LowerSaturationLimit=0.001  ShowSaturationPort=on
  "Powierzchnia dna m  " : Constant  Value=12
  Powierzchnia dna m2 : Constant  Value=12
  "Poziom zbiornik dolny " : Subsystem
  Product : Product  RndMeth=Zero
  Product1 : Product  RndMeth=Zero
  Sat uszk (F>=0)1 : Saturate  UpperLimit=1  LowerLimit=0
  Sum1 : Sum  Inputs=|+-
  Sum2 : Sum  Inputs=|++
  Sum4 : Sum  Inputs=|-+
  Jakosc zacieru brzeczki : Outport
  Gestosc zanieczyszczen : Outport  Port=2
  Przepelnienie : Outport  Port=3
  Poziom wysoki : Outport  Port=4
  Poziom niski : Outport  Port=5
  Temperatura : Outport  Port=6
  Poziom : Outport  Port=7
  wires:
  Sum4/1 -> Objetosc zbiornik dolny/1
  Objetosc zbiornik dolny/1 -> "Poziom zbiornik dolny "/1(Objetosc), Divide1/2, Model jakosci zacieru/1(Objetosc), Model akumulacji ciepla w zbiorniku/1(Objetosc cieczy w zbiorniku)
  Powierzchnia dna m2/1 -> "Poziom zbiornik dolny "/2(Powierzchnia dna)
  Sum1/1 -> Masa zanieczyszczen/1
  Masa zanieczyszczen/1 -> Divide1/1
  Doplyw zanieczyszczen/1 -> Sum1/1
  Divide1/1 -> Gestosc zanieczyszczen/1, Dot Product/2
  "Poziom zbiornik dolny "/1(Poziom  wysoki) -> Poziom wysoki/1
  "Poziom zbiornik dolny "/2(Poziom niski) -> Poziom niski/1
  "Poziom zbiornik dolny "/3(Poziom) -> Poziom/1, Gain/1, Model utratu ciepla/1(Poziom), Display1/1
  Dot Product/1 -> Sum1/2
  Doplyw/1 -> Sum4/2, Model jakosci zacieru/3(Doplyw zacieru), Model akumulacji ciepla w zbiorniku/3(Strumien brzeczki)
  Wyciek/1 -> Sat uszk (F>=0)1/1
  Sat uszk (F>=0)1/1 -> Product/1
  Product1/1 -> Product/2
  Max wyciek/1 -> Product1/1  "m3/s"
  Math Function/1 -> Product1/2
  Gain/1 -> Math Function/1
  Odplyw/1 -> Sum2/1
  Sum2/1 -> Dot Product/1, Sum4/1, Model jakosci zacieru/4(Odplyw), Model akumulacji ciepla w zbiorniku/4(Strumien odplywu cieczy)
  Product/1 -> Sum2/2
  Model jakosci zacieru/1(Jakosc zacieru zbiornika) -> Jakosc zacieru brzeczki/1
  Jakosc zacieru/1 -> Model jakosci zacieru/5(Jakosc zacieru)
  Objetosc zbiornik dolny/2 -> Model jakosci zacieru/2(Przepelnienie), Model akumulacji ciepla w zbiorniku/2(Przepelnienie), Przepelnienie/1
  Model akumulacji ciepla w zbiorniku/1(Temperatura) -> Temperatura/1, Model utratu ciepla/4(Temperatura lustra), Model utratu ciepla/3(Srednia temperatura)
  Temperatura doplywu/1 -> Model akumulacji ciepla w zbiorniku/5(Temperatura strumien doplywu brzeczki)
  Model utratu ciepla/1(Strumien ciepla) -> Model akumulacji ciepla w zbiorniku/6(Strumien ciepla traconego)
  "Powierzchnia dna m  "/1 -> Model utratu ciepla/2(Pole podstawy zbiornika)

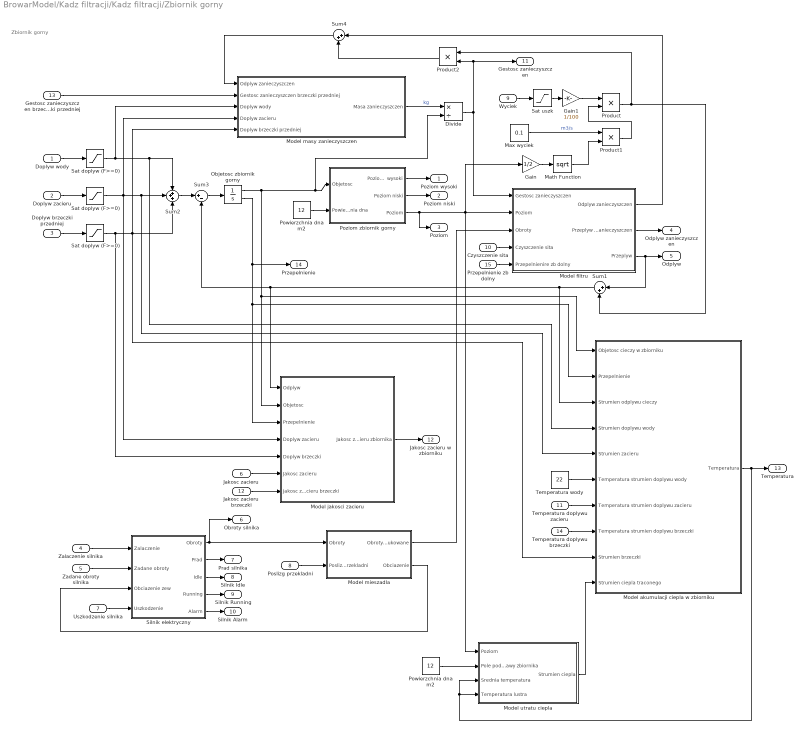
== system BrowarModel/Kadz filtracji/Kadz filtracji/Zbiornik gorny ==
  note: Zbiornik gorny
  Doplyw wody : Inport
  Doplyw zacieru : Inport  Port=2
  Doplyw brzeczki przedniej : Inport  Port=3
  Zalaczenie silnika : Inport  Port=4
  "Zadane obroty silnika " : Inport  Port=5
  Jakosc zacieru : Inport  Port=6
  Uszkodzenie silnika : Inport  Port=7
  Poslizg przekladni : Inport  Port=8
  Wyciek : Inport  Port=9
  Czyszczenie sita : Inport  Port=10
  Temperatura doplywu zacieru : Inport  Port=11
  Jakosc zacieru brzeczki : Inport  Port=12
  Gestosc zanieczyszczen brzeczki przedniej : Inport  Port=13
  Temperatura doplywu brzeczki : Inport  Port=14
  Przepelnienie zb dolny : Inport  Port=15
  Divide : Product  Inputs=*/
  Gain : Gain  Gain=1/2
  Gain1 : Gain  Gain=1/100
  Math Function : Math  Operator=sqrt  SignedPower=on
  Max wyciek : Constant  Value=0.1
  Model akumulacji ciepla w zbiorniku : Subsystem
  Model filtru : Subsystem
  Model jakosci zacieru : Subsystem
  Model masy zanieczyszczen : Subsystem
  Model mieszadla : Subsystem
  Model utratu ciepla : Subsystem
  Objetosc zbiornik gorny : Integrator  InitialCondition=0.001  LimitOutput=on  UpperSaturationLimit=24  LowerSaturationLimit=0.001  ShowSaturationPort=on
  "Powierzchnia dna m2 " : Constant  Value=12
  "Powierzchnia dna m2  " : Constant  Value=12
  "Poziom zbiornik gorny " : Subsystem
  Product : Product  RndMeth=Zero
  Product1 : Product  RndMeth=Zero
  Product2 : Product  RndMeth=Zero
  "Sat doplyw (F>=0)   " : Saturate  UpperLimit=inf  LowerLimit=0
  "Sat doplyw (F>=0) " : Saturate  UpperLimit=inf  LowerLimit=0
  "Sat doplyw (F>=0)  " : Saturate  UpperLimit=inf  LowerLimit=0
  Sat uszk : Saturate  UpperLimit=100  LowerLimit=0
  Silnik elektryczny : Subsystem
  Sum1 : Sum  Inputs=|++
  Sum2 : Sum  Inputs=+++
  Sum3 : Sum  Inputs=|+-
  Sum4 : Sum  Inputs=|++
  Temperatura wody : Constant  Value=22
  Poziom wysoki : Outport
  Poziom niski : Outport  Port=2
  Poziom : Outport  Port=3
  Odplyw zanieczyszczen : Outport  Port=4
  Odplyw : Outport  Port=5
  Obroty silnika : Outport  Port=6
  Prad silnika : Outport  Port=7
  Silnik Idle : Outport  Port=8
  Silnik Running : Outport  Port=9
  Silnik Alarm : Outport  Port=10
  Gestosc zanieczyszczen : Outport  Port=11
  Jakosc zacieru w zbiorniku : Outport  Port=12
  Temperatura : Outport  Port=13
  Przepelnienie : Outport  Port=14
  wires:
  "Sat doplyw (F>=0) "/1 -> Model masy zanieczyszczen/3(Doplyw wody), Sum2/1, Model akumulacji ciepla w zbiorniku/4(Strumien doplywu wody)
  "Sat doplyw (F>=0)  "/1 -> Model masy zanieczyszczen/4(Doplyw zacieru), Model jakosci zacieru/4(Doplyw zacieru), Sum2/2, Model akumulacji ciepla w zbiorniku/5(Strumien zacieru)
  "Sat doplyw (F>=0)   "/1 -> Sum2/3, Model masy zanieczyszczen/5(Doplyw brzeczki przedniej), Model akumulacji ciepla w zbiorniku/9(Strumien brzeczki), Model jakosci zacieru/5(Doplyw brzeczki)
  Sum2/1 -> Sum3/1
  Sum3/1 -> Objetosc zbiornik gorny/1
  Objetosc zbiornik gorny/1 -> Divide/2, "Poziom zbiornik gorny "/1(Objetosc), Model jakosci zacieru/2(Objetosc), Model akumulacji ciepla w zbiorniku/1(Objetosc cieczy w zbiorniku)
  "Powierzchnia dna m2 "/1 -> "Poziom zbiornik gorny "/2(Powierzchnia dna)
  "Poziom zbiornik gorny "/3(Poziom) -> Poziom/1, Model filtru/2(Poziom), Gain/1, Model utratu ciepla/1(Poziom)
  Model filtru/3(Przeplyw) -> Odplyw/1, Sum1/1
  Model masy zanieczyszczen/1(Masa zanieczyszczen) -> Divide/1  "kg"
  Divide/1 -> Model filtru/1(Gestosc zanieczyszczen), Product2/2, Gestosc zanieczyszczen/1
  Gestosc zanieczyszczen brzeczki przedniej/1 -> Model masy zanieczyszczen/2(Gestosc zanieczyszczen brzeczki przedniej)
  Doplyw wody/1 -> "Sat doplyw (F>=0) "/1
  "Poziom zbiornik gorny "/1(Poziom  wysoki) -> Poziom wysoki/1
  Doplyw zacieru/1 -> "Sat doplyw (F>=0)  "/1
  "Poziom zbiornik gorny "/2(Poziom niski) -> Poziom niski/1
  Doplyw brzeczki przedniej/1 -> "Sat doplyw (F>=0)   "/1
  Model filtru/2(Przeplyw zanieczyszczen) -> Odplyw zanieczyszczen/1
  Zalaczenie silnika/1 -> Silnik elektryczny/1(Zalaczenie)
  "Zadane obroty silnika "/1 -> Silnik elektryczny/2(Zadane obroty)
  Uszkodzenie silnika/1 -> Silnik elektryczny/4(Uszkodzenie)
  Model mieszadla/2(Obciazenie) -> Silnik elektryczny/3(Obciazenie zew)
  Poslizg przekladni/1 -> Model mieszadla/2(Poslizg przekladni)
  Model mieszadla/1(Obroty zredukowane) -> Model filtru/3(Obroty)
  Wyciek/1 -> Sat uszk/1
  Sat uszk/1 -> Gain1/1
  Product1/1 -> Product/2
  Max wyciek/1 -> Product1/1  "m3/s"
  Math Function/1 -> Product1/2
  Gain/1 -> Math Function/1
  Sum1/1 -> Sum3/2, Model jakosci zacieru/1(Odplyw), Model akumulacji ciepla w zbiorniku/3(Strumien odplywu cieczy)
  Sum4/1 -> Model masy zanieczyszczen/1(Odplyw zanieczyszczen)
  Model filtru/1(Odplyw zanieczyszczen) -> Sum4/1
  Product2/1 -> Sum4/2
  Product/1 -> Product2/1, Sum1/2
  Objetosc zbiornik gorny/2 -> Model jakosci zacieru/3(Przepelnienie), Model akumulacji ciepla w zbiorniku/2(Przepelnienie), Przepelnienie/1
  Jakosc zacieru/1 -> Model jakosci zacieru/6(Jakosc zacieru)
  Jakosc zacieru brzeczki/1 -> Model jakosci zacieru/7(Jakosc zacieru brzeczki)
  Model jakosci zacieru/1(Jakosc zacieru zbiornika) -> Jakosc zacieru w zbiorniku/1
  Silnik elektryczny/1(Obroty) -> Model mieszadla/1(Obroty), Obroty silnika/1
  Silnik elektryczny/2(Prad) -> Prad silnika/1
  Silnik elektryczny/3(Idle) -> Silnik Idle/1
  Silnik elektryczny/4(Running) -> Silnik Running/1
  Silnik elektryczny/5(Alarm) -> Silnik Alarm/1
  Czyszczenie sita/1 -> Model filtru/4(Czyszczenie sita)
  Gain1/1 -> Product/1
  Model akumulacji ciepla w zbiorniku/1(Temperatura) -> Temperatura/1, Model utratu ciepla/3(Srednia temperatura), Model utratu ciepla/4(Temperatura lustra)
  Temperatura doplywu zacieru/1 -> Model akumulacji ciepla w zbiorniku/7(Temperatura strumien doplywu zacieru)
  Temperatura wody/1 -> Model akumulacji ciepla w zbiorniku/6(Temperatura strumien doplywu wody)
  Temperatura doplywu brzeczki/1 -> Model akumulacji ciepla w zbiorniku/8(Temperatura strumien doplywu brzeczki)
  Model utratu ciepla/1(Strumien ciepla) -> Model akumulacji ciepla w zbiorniku/10(Strumien ciepla traconego)
  "Powierzchnia dna m2  "/1 -> Model utratu ciepla/2(Pole podstawy zbiornika)
  Przepelnienie zb dolny/1 -> Model filtru/5(Przepelnienire zb dolny)

== system BrowarModel/Kadz filtracji/LT308/Zaklocenia pomiarowe ==
  Product1 : Product  InputSameDT=on  RndMeth=Zero  SaturateOnIntegerOverflow=on  OutDataTypeStr=Inherit: Same as first input
  Product3 : Product  InputSameDT=on  RndMeth=Zero  SaturateOnIntegerOverflow=on  OutDataTypeStr=Inherit: Same as first input
  Random Number : RandomNumber  Variance=.5  Seed=4365624  SampleTime=0.1
  Transfer Fcn1 : TransferFcn  Denominator=[0.5 1]
  Transfer Fcn2 : TransferFcn  Denominator=[0.5 1]
  Zaklocenia pomiarowe : Constant  Value=ZakloceniaPom
  Out : Outport
  wires:
  Product1/1 -> Product3/2
  [ZaklPom] -> Product1/1
  Zaklocenia pomiarowe/1 -> Product1/2
  Transfer Fcn2/1 -> Out/1
  Transfer Fcn1/1 -> Transfer Fcn2/1
  Product3/1 -> Transfer Fcn1/1
  Random Number/1 -> Product3/1

== system BrowarModel/Kadz filtracji/LT309/Zaklocenia pomiarowe ==
  Product1 : Product  InputSameDT=on  RndMeth=Zero  SaturateOnIntegerOverflow=on  OutDataTypeStr=Inherit: Same as first input
  Product3 : Product  InputSameDT=on  RndMeth=Zero  SaturateOnIntegerOverflow=on  OutDataTypeStr=Inherit: Same as first input
  Random Number : RandomNumber  Variance=.5  Seed=4365624  SampleTime=0.1
  Transfer Fcn1 : TransferFcn  Denominator=[0.5 1]
  Transfer Fcn2 : TransferFcn  Denominator=[0.5 1]
  Zaklocenia pomiarowe : Constant  Value=ZakloceniaPom
  Out : Outport
  wires:
  Random Number/1 -> Product3/1
  Product3/1 -> Transfer Fcn1/1
  Transfer Fcn1/1 -> Transfer Fcn2/1
  Transfer Fcn2/1 -> Out/1
  Zaklocenia pomiarowe/1 -> Product1/2
  [ZaklPom] -> Product1/1
  Product1/1 -> Product3/2

== system BrowarModel/Kadz filtracji/QT310/Zaklocenia pomiarowe ==
  Product1 : Product  InputSameDT=on  RndMeth=Zero  SaturateOnIntegerOverflow=on  OutDataTypeStr=Inherit: Same as first input
  Product3 : Product  InputSameDT=on  RndMeth=Zero  SaturateOnIntegerOverflow=on  OutDataTypeStr=Inherit: Same as first input
  Random Number : RandomNumber  Variance=.5  Seed=4365624  SampleTime=0.1
  Transfer Fcn1 : TransferFcn  Denominator=[0.5 1]
  Transfer Fcn2 : TransferFcn  Denominator=[0.5 1]
  Zaklocenia pomiarowe : Constant  Value=ZakloceniaPom
  Out : Outport
  wires:
  Random Number/1 -> Product3/1
  Product3/1 -> Transfer Fcn1/1
  Transfer Fcn1/1 -> Transfer Fcn2/1
  Transfer Fcn2/1 -> Out/1
  Zaklocenia pomiarowe/1 -> Product1/2
  [ZaklPom] -> Product1/1
  Product1/1 -> Product3/2

== system BrowarModel/Kadz filtracji/QT311/Zaklocenia pomiarowe ==
  Product1 : Product  InputSameDT=on  RndMeth=Zero  SaturateOnIntegerOverflow=on  OutDataTypeStr=Inherit: Same as first input
  Product3 : Product  InputSameDT=on  RndMeth=Zero  SaturateOnIntegerOverflow=on  OutDataTypeStr=Inherit: Same as first input
  Random Number : RandomNumber  Variance=.5  Seed=4365624  SampleTime=0.1
  Transfer Fcn1 : TransferFcn  Denominator=[0.5 1]
  Transfer Fcn2 : TransferFcn  Denominator=[0.5 1]
  Zaklocenia pomiarowe : Constant  Value=ZakloceniaPom
  Out : Outport
  wires:
  Product1/1 -> Product3/2
  [ZaklPom] -> Product1/1
  Zaklocenia pomiarowe/1 -> Product1/2
  Transfer Fcn2/1 -> Out/1
  Transfer Fcn1/1 -> Transfer Fcn2/1
  Product3/1 -> Transfer Fcn1/1
  Random Number/1 -> Product3/1

== system BrowarModel/Kadz filtracji/QT312/Zaklocenia pomiarowe ==
  Product1 : Product  InputSameDT=on  RndMeth=Zero  SaturateOnIntegerOverflow=on  OutDataTypeStr=Inherit: Same as first input
  Product3 : Product  InputSameDT=on  RndMeth=Zero  SaturateOnIntegerOverflow=on  OutDataTypeStr=Inherit: Same as first input
  Random Number : RandomNumber  Variance=.5  Seed=4365624  SampleTime=0.1
  Transfer Fcn1 : TransferFcn  Denominator=[0.5 1]
  Transfer Fcn2 : TransferFcn  Denominator=[0.5 1]
  Zaklocenia pomiarowe : Constant  Value=ZakloceniaPom
  Out : Outport
  wires:
  Random Number/1 -> Product3/1
  Product3/1 -> Transfer Fcn1/1
  Transfer Fcn1/1 -> Transfer Fcn2/1
  Transfer Fcn2/1 -> Out/1
  Zaklocenia pomiarowe/1 -> Product1/2
  [ZaklPom] -> Product1/1
  Product1/1 -> Product3/2

== system BrowarModel/Kadz filtracji/ST302/Zaklocenia pomiarowe ==
  Product1 : Product  InputSameDT=on  RndMeth=Zero  SaturateOnIntegerOverflow=on  OutDataTypeStr=Inherit: Same as first input
  Product3 : Product  InputSameDT=on  RndMeth=Zero  SaturateOnIntegerOverflow=on  OutDataTypeStr=Inherit: Same as first input
  Random Number : RandomNumber  Variance=.5  Seed=4365624  SampleTime=0.1
  Transfer Fcn1 : TransferFcn  Denominator=[0.5 1]
  Transfer Fcn2 : TransferFcn  Denominator=[0.5 1]
  Zaklocenia pomiarowe : Constant  Value=ZakloceniaPom
  Out : Outport
  wires:
  Product1/1 -> Product3/2
  [ZaklPom] -> Product1/1
  Zaklocenia pomiarowe/1 -> Product1/2
  Transfer Fcn2/1 -> Out/1
  Transfer Fcn1/1 -> Transfer Fcn2/1
  Product3/1 -> Transfer Fcn1/1
  Random Number/1 -> Product3/1

== system BrowarModel/Kadz filtracji/ST304/Zaklocenia pomiarowe ==
  Product1 : Product  InputSameDT=on  RndMeth=Zero  SaturateOnIntegerOverflow=on  OutDataTypeStr=Inherit: Same as first input
  Product3 : Product  InputSameDT=on  RndMeth=Zero  SaturateOnIntegerOverflow=on  OutDataTypeStr=Inherit: Same as first input
  Random Number : RandomNumber  Variance=.5  Seed=4365624  SampleTime=0.1
  Transfer Fcn1 : TransferFcn  Denominator=[0.5 1]
  Transfer Fcn2 : TransferFcn  Denominator=[0.5 1]
  Zaklocenia pomiarowe : Constant  Value=ZakloceniaPom
  Out : Outport
  wires:
  Random Number/1 -> Product3/1
  Product3/1 -> Transfer Fcn1/1
  Transfer Fcn1/1 -> Transfer Fcn2/1
  Transfer Fcn2/1 -> Out/1
  Zaklocenia pomiarowe/1 -> Product1/2
  [ZaklPom] -> Product1/1
  Product1/1 -> Product3/2

== system BrowarModel/Kadz filtracji/ST307/Zaklocenia pomiarowe ==
  Product1 : Product  InputSameDT=on  RndMeth=Zero  SaturateOnIntegerOverflow=on  OutDataTypeStr=Inherit: Same as first input
  Product3 : Product  InputSameDT=on  RndMeth=Zero  SaturateOnIntegerOverflow=on  OutDataTypeStr=Inherit: Same as first input
  Random Number : RandomNumber  Variance=.5  Seed=4365624  SampleTime=0.1
  Transfer Fcn1 : TransferFcn  Denominator=[0.5 1]
  Transfer Fcn2 : TransferFcn  Denominator=[0.5 1]
  Zaklocenia pomiarowe : Constant  Value=ZakloceniaPom
  Out : Outport
  wires:
  Random Number/1 -> Product3/1
  Product3/1 -> Transfer Fcn1/1
  Transfer Fcn1/1 -> Transfer Fcn2/1
  Transfer Fcn2/1 -> Out/1
  Zaklocenia pomiarowe/1 -> Product1/2
  [ZaklPom] -> Product1/1
  Product1/1 -> Product3/2

== system BrowarModel/Kadz warzelna/ET404/Zaklocenia pomiarowe ==
  Product1 : Product  InputSameDT=on  RndMeth=Zero  SaturateOnIntegerOverflow=on  OutDataTypeStr=Inherit: Same as first input
  Product3 : Product  InputSameDT=on  RndMeth=Zero  SaturateOnIntegerOverflow=on  OutDataTypeStr=Inherit: Same as first input
  Random Number : RandomNumber  Variance=.5  Seed=4365624  SampleTime=0.1
  Transfer Fcn1 : TransferFcn  Denominator=[0.5 1]
  Transfer Fcn2 : TransferFcn  Denominator=[0.5 1]
  Zaklocenia pomiarowe : Constant  Value=ZakloceniaPom
  Out : Outport
  wires:
  Random Number/1 -> Product3/1
  Product3/1 -> Transfer Fcn1/1
  Transfer Fcn1/1 -> Transfer Fcn2/1
  Transfer Fcn2/1 -> Out/1
  Zaklocenia pomiarowe/1 -> Product1/2
  [ZaklPom] -> Product1/1
  Product1/1 -> Product3/2
